simulink model "top_level_arch"  (R2025b)
settings: Solver=VariableStepAuto  StartTime=0.0  StopTime=10.0  RelTol=1e-3
undefined symbols (not defined in the file): D, L
(part 2 of 2)

== system top_level_arch/Manufacturing /Available Components/Propulsion ==
  Technology : Inport
  Supply Chain : Inport  Port=2
  Liquid Rocket : Subsystem  VariantControl=Ramjet1
      settings: PortSchema="{\"entries\":[{\"content\":{\"headerSize\":26,\"margin\":15,\"minimumSpacing\":25,\"sides\":[{\"content\":{},\"type\":\"ConnectorPlacement.EquallySpacedRectSide\",\"uuid\":\"e5d1d625-0a19-4884-bba9-d999bfe05807\"},{\"content\":{\"side\":\"RIGHT\"},\"type\":\"ConnectorPlacement.EquallySpacedRectSide\",\"uuid\":\"e3bc6884-47ae-4782-b1b3-7f6467d3ceaa\"},{\"content\":{\"side\":\"TOP\"},\"type\":\"ConnectorPlacement.EquallySpacedRectSide\",\"uuid\":\"e69a1f27-d2d1-47d9-a5bf-aefa7bba6fe5\"}]},\"type\":\"ConnectorPlacement.EquallySpacedConnector\",\"uuid\":\"2d31618d-9212-4cde-94a4-f40aa24b68df\"}],\"packageUris\":[\"http://schema.mathworks.com/mf0/Connector/R2020b\"],\"version\":\"1.0\"}"
  RDRE : Subsystem  VariantControl=true
      settings: PortSchema="{\"entries\":[{\"content\":{\"headerSize\":26,\"margin\":15,\"minimumSpacing\":25,\"sides\":[{\"content\":{},\"type\":\"ConnectorPlacement.EquallySpacedRectSide\",\"uuid\":\"e5d1d625-0a19-4884-bba9-d999bfe05807\"},{\"content\":{\"side\":\"RIGHT\"},\"type\":\"ConnectorPlacement.EquallySpacedRectSide\",\"uuid\":\"e3bc6884-47ae-4782-b1b3-7f6467d3ceaa\"},{\"content\":{\"side\":\"TOP\"},\"type\":\"ConnectorPlacement.EquallySpacedRectSide\",\"uuid\":\"e69a1f27-d2d1-47d9-a5bf-aefa7bba6fe5\"}]},\"type\":\"ConnectorPlacement.EquallySpacedConnector\",\"uuid\":\"2d31618d-9212-4cde-94a4-f40aa24b68df\"}],\"packageUris\":[\"http://schema.mathworks.com/mf0/Connector/R2020b\"],\"version\":\"1.0\"}"
  Ramjet : Subsystem  VariantControl=Turbojet1
      settings: PortSchema="{\"entries\":[{\"content\":{\"headerSize\":26,\"margin\":15,\"minimumSpacing\":25,\"sides\":[{\"content\":{},\"type\":\"ConnectorPlacement.EquallySpacedRectSide\",\"uuid\":\"e5d1d625-0a19-4884-bba9-d999bfe05807\"},{\"content\":{\"side\":\"RIGHT\"},\"type\":\"ConnectorPlacement.EquallySpacedRectSide\",\"uuid\":\"e3bc6884-47ae-4782-b1b3-7f6467d3ceaa\"},{\"content\":{\"side\":\"TOP\"},\"type\":\"ConnectorPlacement.EquallySpacedRectSide\",\"uuid\":\"e69a1f27-d2d1-47d9-a5bf-aefa7bba6fe5\"}]},\"type\":\"ConnectorPlacement.EquallySpacedConnector\",\"uuid\":\"2d31618d-9212-4cde-94a4-f40aa24b68df\"}],\"packageUris\":[\"http://schema.mathworks.com/mf0/Connector/R2020b\"],\"version\":\"1.0\"}"
  Solid Rocket : Subsystem  VariantControl=Liquid Rocket1
      settings: PortSchema="{\"entries\":[{\"content\":{\"headerSize\":26,\"margin\":15,\"minimumSpacing\":25,\"sides\":[{\"content\":{},\"type\":\"ConnectorPlacement.EquallySpacedRectSide\",\"uuid\":\"e5d1d625-0a19-4884-bba9-d999bfe05807\"},{\"content\":{\"side\":\"RIGHT\"},\"type\":\"ConnectorPlacement.EquallySpacedRectSide\",\"uuid\":\"e3bc6884-47ae-4782-b1b3-7f6467d3ceaa\"},{\"content\":{\"side\":\"TOP\"},\"type\":\"ConnectorPlacement.EquallySpacedRectSide\",\"uuid\":\"e69a1f27-d2d1-47d9-a5bf-aefa7bba6fe5\"}]},\"type\":\"ConnectorPlacement.EquallySpacedConnector\",\"uuid\":\"2d31618d-9212-4cde-94a4-f40aa24b68df\"}],\"packageUris\":[\"http://schema.mathworks.com/mf0/Connector/R2020b\"],\"version\":\"1.0\"}"
  Turbojet : Subsystem  VariantControl=false
      settings: PortSchema="{\"entries\":[{\"content\":{\"headerSize\":26,\"margin\":15,\"minimumSpacing\":25,\"sides\":[{\"content\":{},\"type\":\"ConnectorPlacement.EquallySpacedRectSide\",\"uuid\":\"e5d1d625-0a19-4884-bba9-d999bfe05807\"},{\"content\":{\"side\":\"RIGHT\"},\"type\":\"ConnectorPlacement.EquallySpacedRectSide\",\"uuid\":\"e3bc6884-47ae-4782-b1b3-7f6467d3ceaa\"},{\"content\":{\"side\":\"TOP\"},\"type\":\"ConnectorPlacement.EquallySpacedRectSide\",\"uuid\":\"e69a1f27-d2d1-47d9-a5bf-aefa7bba6fe5\"}]},\"type\":\"ConnectorPlacement.EquallySpacedConnector\",\"uuid\":\"2d31618d-9212-4cde-94a4-f40aa24b68df\"}],\"packageUris\":[\"http://schema.mathworks.com/mf0/Connector/R2020b\"],\"version\":\"1.0\"}"
  Propulsion Selection : Outport

== system top_level_arch/Manufacturing /Available Components/Software ==
  Bus Element In1 : Inport  PortName=Technology
  Bus Element In2 : Inport  Port=2  PortName=Supply Chain
  Bus Element Out1 : Outport  PortName=Software Vendor

== system top_level_arch/Scorpius Missile/Aerodynamics/Cylindrical ==

== system top_level_arch/Scorpius Missile/Aerodynamics/Delta Wing ==

== system top_level_arch/Scorpius Missile/Aerodynamics/Lifting Body ==

== system top_level_arch/Scorpius Missile/Configuration/External Hull ==
  Bus Element In1 : Inport  PortName=Assembly
  Bus Element Out1 : Outport  PortName=External Volume

== system top_level_arch/Scorpius Missile/Configuration/Folding Surfaces ==
  Assembly : Inport
  Folding Wings + Fins : Subsystem  VariantControl=false
      settings: PortSchema="{\"entries\":[{\"content\":{\"headerSize\":26,\"margin\":15,\"minimumSpacing\":25,\"sides\":[{\"content\":{},\"type\":\"ConnectorPlacement.EquallySpacedRectSide\",\"uuid\":\"ac629711-1768-428b-8fd7-79e4fe2b35a1\"},{\"content\":{\"side\":\"RIGHT\"},\"type\":\"ConnectorPlacement.EquallySpacedRectSide\",\"uuid\":\"b9c43ceb-249f-4c48-950c-a08a709e2313\"},{\"content\":{\"side\":\"TOP\"},\"type\":\"ConnectorPlacement.EquallySpacedRectSide\",\"uuid\":\"78a92a70-2dde-432d-9083-f129ee7bb076\"}]},\"type\":\"ConnectorPlacement.EquallySpacedConnector\",\"uuid\":\"b2b722ac-28c2-40e7-82d5-b0c5abc634fd\"}],\"packageUris\":[\"http://schema.mathworks.com/mf0/Connector/R2020b\"],\"version\":\"1.0\"}"
  Folding X-Fin : Subsystem  VariantControl=true
      settings: PortSchema="{\"entries\":[{\"content\":{\"headerSize\":26,\"margin\":15,\"minimumSpacing\":25,\"sides\":[{\"content\":{},\"type\":\"ConnectorPlacement.EquallySpacedRectSide\",\"uuid\":\"ac629711-1768-428b-8fd7-79e4fe2b35a1\"},{\"content\":{\"side\":\"RIGHT\"},\"type\":\"ConnectorPlacement.EquallySpacedRectSide\",\"uuid\":\"b9c43ceb-249f-4c48-950c-a08a709e2313\"},{\"content\":{\"side\":\"TOP\"},\"type\":\"ConnectorPlacement.EquallySpacedRectSide\",\"uuid\":\"78a92a70-2dde-432d-9083-f129ee7bb076\"}]},\"type\":\"ConnectorPlacement.EquallySpacedConnector\",\"uuid\":\"b2b722ac-28c2-40e7-82d5-b0c5abc634fd\"}],\"packageUris\":[\"http://schema.mathworks.com/mf0/Connector/R2020b\"],\"version\":\"1.0\"}"
  Launch Volume : Outport

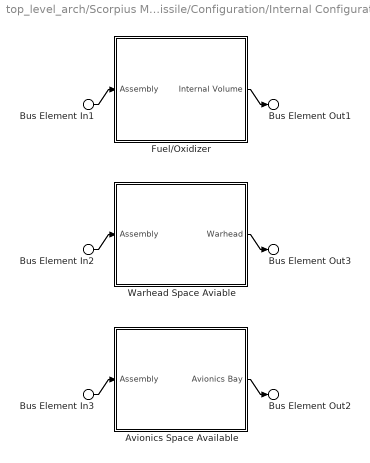
== system top_level_arch/Scorpius Missile/Configuration/Internal Configuration ==
  Bus Element In1 : Inport  PortName=Assembly
  Bus Element In2 : Inport  PortName=Assembly
  Bus Element In3 : Inport  PortName=Assembly
  Avionics Space Available : Subsystem
      settings: PortSchema="{\"entries\":[{\"content\":{\"headerSize\":26,\"margin\":15,\"minimumSpacing\":25,\"sides\":[{\"content\":{\"connectorIds\":[\"In1\"]},\"type\":\"ConnectorPlacement.EquallySpacedRectSide\",\"uuid\":\"dbfe6f62-bd81-4f2f-bf4a-ff0fc2c1733e\"},{\"content\":{\"connectorIds\":[\"Out1\"],\"side\":\"RIGHT\"},\"type\":\"ConnectorPlacement.EquallySpacedRectSide\",\"uuid\":\"15bb1ddd-14b3-4afc-89a1-8972fd4dab01\"},{\"content\":{\"side\":\"TOP\"},\"type\":\"ConnectorPlacement.EquallySpacedRectSide\",\"uuid\":\"d6068651-eb1a-4d26-9e8b-0135dded722b\"}]},\"type\":\"ConnectorPlacement.EquallySpacedConnector\",\"uuid\":\"074be2fd-c315-4aa4-8fc0-0402952ab401\"}],\"packageUris\":[\"http://schema.mathworks.com/mf0/Connector/R2020b\"],\"version\":\"1.0\"}"
  Fuel/Oxidizer : Subsystem
      settings: PortSchema="{\"entries\":[{\"content\":{\"headerSize\":26,\"margin\":15,\"minimumSpacing\":25,\"sides\":[{\"content\":{\"connectorIds\":[\"In1\"]},\"type\":\"ConnectorPlacement.EquallySpacedRectSide\",\"uuid\":\"dbfe6f62-bd81-4f2f-bf4a-ff0fc2c1733e\"},{\"content\":{\"connectorIds\":[\"Out1\"],\"side\":\"RIGHT\"},\"type\":\"ConnectorPlacement.EquallySpacedRectSide\",\"uuid\":\"15bb1ddd-14b3-4afc-89a1-8972fd4dab01\"},{\"content\":{\"side\":\"TOP\"},\"type\":\"ConnectorPlacement.EquallySpacedRectSide\",\"uuid\":\"d6068651-eb1a-4d26-9e8b-0135dded722b\"}]},\"type\":\"ConnectorPlacement.EquallySpacedConnector\",\"uuid\":\"074be2fd-c315-4aa4-8fc0-0402952ab401\"}],\"packageUris\":[\"http://schema.mathworks.com/mf0/Connector/R2020b\"],\"version\":\"1.0\"}"
  Warhead Space Aviable : Subsystem
      settings: PortSchema="{\"entries\":[{\"content\":{\"headerSize\":26,\"margin\":15,\"minimumSpacing\":25,\"sides\":[{\"content\":{\"connectorIds\":[\"In1\"]},\"type\":\"ConnectorPlacement.EquallySpacedRectSide\",\"uuid\":\"dbfe6f62-bd81-4f2f-bf4a-ff0fc2c1733e\"},{\"content\":{\"connectorIds\":[\"Out1\"],\"side\":\"RIGHT\"},\"type\":\"ConnectorPlacement.EquallySpacedRectSide\",\"uuid\":\"15bb1ddd-14b3-4afc-89a1-8972fd4dab01\"},{\"content\":{\"side\":\"TOP\"},\"type\":\"ConnectorPlacement.EquallySpacedRectSide\",\"uuid\":\"d6068651-eb1a-4d26-9e8b-0135dded722b\"}]},\"type\":\"ConnectorPlacement.EquallySpacedConnector\",\"uuid\":\"074be2fd-c315-4aa4-8fc0-0402952ab401\"}],\"packageUris\":[\"http://schema.mathworks.com/mf0/Connector/R2020b\"],\"version\":\"1.0\"}"
  Bus Element Out1 : Outport  PortName=Internal Volume
  Bus Element Out3 : Outport  Port=2  PortName=Warhead
  Bus Element Out2 : Outport  Port=3  PortName=Avionics Bay
  wires:
  Bus Element In1/1 -> Fuel/Oxidizer/1(Assembly)
  Bus Element In2/1 -> Warhead Space Aviable/1(Assembly)
  Bus Element In3/1 -> Avionics Space Available/1(Assembly)
  Fuel/Oxidizer/1(Internal Volume) -> Bus Element Out1/1
  Warhead Space Aviable/1(Warhead) -> Bus Element Out3/1
  Avionics Space Available/1(Avionics Bay) -> Bus Element Out2/1

== system top_level_arch/Scorpius Missile/Propulsion/Fuel//Oxidizer Tank ==
  Bus Element In1 : Inport  PortName=Internal Volume
  Bus Element Out1 : Outport  PortName=Fuel Capacity

== system top_level_arch/Scorpius Missile/Propulsion/RDRE ==
  Bus Element In1 : Inport  PortName=Fuel Capacity
  Bus Element Out2 : Outport  PortName=Supersonic Cruise
  Bus Element Out1 : Outport  Port=2  PortName=Fuel Consumption
  Bus Element Out3 : Outport  Port=3  PortName=Thrust

== system top_level_arch/Scorpius Missile/Trajectory/Approach ==
  Avionics Bay : Inport
  L/D : Inport  Port=2
  Range : Inport  Port=3
  Direct Dive : Subsystem  VariantControl=true  mask{DiveRange=[]}
      settings: PortSchema="{\"entries\":[{\"content\":{\"headerSize\":26,\"margin\":15,\"minimumSpacing\":25,\"sides\":[{\"content\":{},\"type\":\"ConnectorPlacement.EquallySpacedRectSide\",\"uuid\":\"ac629711-1768-428b-8fd7-79e4fe2b35a1\"},{\"content\":{\"side\":\"RIGHT\"},\"type\":\"ConnectorPlacement.EquallySpacedRectSide\",\"uuid\":\"b9c43ceb-249f-4c48-950c-a08a709e2313\"},{\"content\":{\"side\":\"TOP\"},\"type\":\"ConnectorPlacement.EquallySpacedRectSide\",\"uuid\":\"78a92a70-2dde-432d-9083-f129ee7bb076\"}]},\"type\":\"ConnectorPlacement.EquallySpacedConnector\",\"uuid\":\"b2b722ac-28c2-40e7-82d5-b0c5abc634fd\"}],\"packageUris\":[\"http://schema.mathworks.com/mf0/Connector/R2020b\"],\"version\":\"1.0\"}"
  Low Level Ingress : Subsystem  VariantControl=false  mask{LLIRange=[]}
      settings: PortSchema="{\"entries\":[{\"content\":{\"headerSize\":26,\"margin\":15,\"minimumSpacing\":25,\"sides\":[{\"content\":{},\"type\":\"ConnectorPlacement.EquallySpacedRectSide\",\"uuid\":\"ac629711-1768-428b-8fd7-79e4fe2b35a1\"},{\"content\":{\"side\":\"RIGHT\"},\"type\":\"ConnectorPlacement.EquallySpacedRectSide\",\"uuid\":\"b9c43ceb-249f-4c48-950c-a08a709e2313\"},{\"content\":{\"side\":\"TOP\"},\"type\":\"ConnectorPlacement.EquallySpacedRectSide\",\"uuid\":\"78a92a70-2dde-432d-9083-f129ee7bb076\"}]},\"type\":\"ConnectorPlacement.EquallySpacedConnector\",\"uuid\":\"b2b722ac-28c2-40e7-82d5-b0c5abc634fd\"}],\"packageUris\":[\"http://schema.mathworks.com/mf0/Connector/R2020b\"],\"version\":\"1.0\"}"
  Approach Phase : Outport
  Target Approach : Outport  Port=2

== system top_level_arch/Scorpius Missile/Trajectory/Climb ==
  Bus Element In1 : Inport  PortName=L/D
  Bus Element In2 : Inport  Port=2  PortName=Range
  Bus Element In3 : Inport  Port=3  PortName=Thrust
  Bus Element Out1 : Outport  PortName=Climb Phase

== system top_level_arch/Scorpius Missile/Trajectory/Cruise ==
  Bus Element In1 : Inport  PortName=L/D
  Bus Element In2 : Inport  Port=2  PortName=Range
  Bus Element In3 : Inport  Port=3  PortName=Thrust
  Bus Element Out1 : Outport  PortName=Cruise Phase

== system top_level_arch/Scorpius Missile/Trajectory/Glide ==
  Bus Element In1 : Inport  PortName=L/D
  Bus Element Out1 : Outport  PortName=Glide Phase

== system top_level_arch/Manufacturing /Available Components/Avionics Package/Air Data System ==
  Technology : Inport
  Supply Chain : Inport  Port=2
  Flush Air Data System : Subsystem  VariantControl=false
      settings: PortSchema="{\"entries\":[{\"content\":{\"headerSize\":26,\"margin\":15,\"minimumSpacing\":25,\"sides\":[{\"content\":{},\"type\":\"ConnectorPlacement.EquallySpacedRectSide\",\"uuid\":\"ac629711-1768-428b-8fd7-79e4fe2b35a1\"},{\"content\":{\"side\":\"RIGHT\"},\"type\":\"ConnectorPlacement.EquallySpacedRectSide\",\"uuid\":\"b9c43ceb-249f-4c48-950c-a08a709e2313\"},{\"content\":{\"side\":\"TOP\"},\"type\":\"ConnectorPlacement.EquallySpacedRectSide\",\"uuid\":\"78a92a70-2dde-432d-9083-f129ee7bb076\"}]},\"type\":\"ConnectorPlacement.EquallySpacedConnector\",\"uuid\":\"b2b722ac-28c2-40e7-82d5-b0c5abc634fd\"}],\"packageUris\":[\"http://schema.mathworks.com/mf0/Connector/R2020b\"],\"version\":\"1.0\"}"
  Pitot Tube : Subsystem  VariantControl=true
      settings: PortSchema="{\"entries\":[{\"content\":{\"headerSize\":26,\"margin\":15,\"minimumSpacing\":25,\"sides\":[{\"content\":{},\"type\":\"ConnectorPlacement.EquallySpacedRectSide\",\"uuid\":\"ac629711-1768-428b-8fd7-79e4fe2b35a1\"},{\"content\":{\"side\":\"RIGHT\"},\"type\":\"ConnectorPlacement.EquallySpacedRectSide\",\"uuid\":\"b9c43ceb-249f-4c48-950c-a08a709e2313\"},{\"content\":{\"side\":\"TOP\"},\"type\":\"ConnectorPlacement.EquallySpacedRectSide\",\"uuid\":\"78a92a70-2dde-432d-9083-f129ee7bb076\"}]},\"type\":\"ConnectorPlacement.EquallySpacedConnector\",\"uuid\":\"b2b722ac-28c2-40e7-82d5-b0c5abc634fd\"}],\"packageUris\":[\"http://schema.mathworks.com/mf0/Connector/R2020b\"],\"version\":\"1.0\"}"
  Air Data Selection : Outport

== system top_level_arch/Manufacturing /Available Components/Avionics Package/Battery ==
  Technology : Inport
  Supply Chain : Inport  Port=2
  Battery 1 : Subsystem  VariantControl=true
      settings: PortSchema="{\"entries\":[{\"content\":{\"headerSize\":26,\"margin\":15,\"minimumSpacing\":25,\"sides\":[{\"content\":{},\"type\":\"ConnectorPlacement.EquallySpacedRectSide\",\"uuid\":\"ac629711-1768-428b-8fd7-79e4fe2b35a1\"},{\"content\":{\"side\":\"RIGHT\"},\"type\":\"ConnectorPlacement.EquallySpacedRectSide\",\"uuid\":\"b9c43ceb-249f-4c48-950c-a08a709e2313\"},{\"content\":{\"side\":\"TOP\"},\"type\":\"ConnectorPlacement.EquallySpacedRectSide\",\"uuid\":\"78a92a70-2dde-432d-9083-f129ee7bb076\"}]},\"type\":\"ConnectorPlacement.EquallySpacedConnector\",\"uuid\":\"b2b722ac-28c2-40e7-82d5-b0c5abc634fd\"}],\"packageUris\":[\"http://schema.mathworks.com/mf0/Connector/R2020b\"],\"version\":\"1.0\"}"
  Battery 2 : Subsystem  VariantControl=false
      settings: PortSchema="{\"entries\":[{\"content\":{\"headerSize\":26,\"margin\":15,\"minimumSpacing\":25,\"sides\":[{\"content\":{},\"type\":\"ConnectorPlacement.EquallySpacedRectSide\",\"uuid\":\"ac629711-1768-428b-8fd7-79e4fe2b35a1\"},{\"content\":{\"side\":\"RIGHT\"},\"type\":\"ConnectorPlacement.EquallySpacedRectSide\",\"uuid\":\"b9c43ceb-249f-4c48-950c-a08a709e2313\"},{\"content\":{\"side\":\"TOP\"},\"type\":\"ConnectorPlacement.EquallySpacedRectSide\",\"uuid\":\"78a92a70-2dde-432d-9083-f129ee7bb076\"}]},\"type\":\"ConnectorPlacement.EquallySpacedConnector\",\"uuid\":\"b2b722ac-28c2-40e7-82d5-b0c5abc634fd\"}],\"packageUris\":[\"http://schema.mathworks.com/mf0/Connector/R2020b\"],\"version\":\"1.0\"}"
  Battery Selection : Outport

== system top_level_arch/Manufacturing /Available Components/Avionics Package/Guidance Package ==
  Target Approach : Inport
  Technology : Inport  Port=2
  Supply Chain : Inport  Port=3
  Dive Package : Subsystem  VariantControl=true
      settings: PortSchema="{\"entries\":[{\"content\":{\"headerSize\":26,\"margin\":15,\"minimumSpacing\":25,\"sides\":[{\"content\":{},\"type\":\"ConnectorPlacement.EquallySpacedRectSide\",\"uuid\":\"ac629711-1768-428b-8fd7-79e4fe2b35a1\"},{\"content\":{\"side\":\"RIGHT\"},\"type\":\"ConnectorPlacement.EquallySpacedRectSide\",\"uuid\":\"b9c43ceb-249f-4c48-950c-a08a709e2313\"},{\"content\":{\"side\":\"TOP\"},\"type\":\"ConnectorPlacement.EquallySpacedRectSide\",\"uuid\":\"78a92a70-2dde-432d-9083-f129ee7bb076\"}]},\"type\":\"ConnectorPlacement.EquallySpacedConnector\",\"uuid\":\"b2b722ac-28c2-40e7-82d5-b0c5abc634fd\"}],\"packageUris\":[\"http://schema.mathworks.com/mf0/Connector/R2020b\"],\"version\":\"1.0\"}"
  LLI Package : Subsystem  VariantControl=false
      settings: PortSchema="{\"entries\":[{\"content\":{\"headerSize\":26,\"margin\":15,\"minimumSpacing\":25,\"sides\":[{\"content\":{},\"type\":\"ConnectorPlacement.EquallySpacedRectSide\",\"uuid\":\"ac629711-1768-428b-8fd7-79e4fe2b35a1\"},{\"content\":{\"side\":\"RIGHT\"},\"type\":\"ConnectorPlacement.EquallySpacedRectSide\",\"uuid\":\"b9c43ceb-249f-4c48-950c-a08a709e2313\"},{\"content\":{\"side\":\"TOP\"},\"type\":\"ConnectorPlacement.EquallySpacedRectSide\",\"uuid\":\"78a92a70-2dde-432d-9083-f129ee7bb076\"}]},\"type\":\"ConnectorPlacement.EquallySpacedConnector\",\"uuid\":\"b2b722ac-28c2-40e7-82d5-b0c5abc634fd\"}],\"packageUris\":[\"http://schema.mathworks.com/mf0/Connector/R2020b\"],\"version\":\"1.0\"}"
  Guidance Selection : Outport

== system top_level_arch/Manufacturing /Available Components/Avionics Package/Target Identification//Tracking ==
  Bus Element In1 : Inport  PortName=Technology
  Bus Element In2 : Inport  Port=2  PortName=Supply Chain
  IR Camera : Subsystem
      settings: PortSchema="{\"entries\":[{\"content\":{\"headerSize\":26,\"margin\":15,\"minimumSpacing\":25,\"sides\":[{\"content\":{},\"type\":\"ConnectorPlacement.EquallySpacedRectSide\",\"uuid\":\"acffec25-5f7e-46a6-bfc3-7ef631e1638e\"},{\"content\":{\"side\":\"RIGHT\"},\"type\":\"ConnectorPlacement.EquallySpacedRectSide\",\"uuid\":\"2e9e2c31-11a0-4694-98ae-75af4a65f270\"},{\"content\":{\"side\":\"TOP\"},\"type\":\"ConnectorPlacement.EquallySpacedRectSide\",\"uuid\":\"496cd80b-0660-4c9b-9e86-ee3459eee66e\"}]},\"type\":\"ConnectorPlacement.EquallySpacedConnector\",\"uuid\":\"b09bcaf7-bc67-4c5f-bdb5-a74881794e47\"}],\"packageUris\":[\"http://schema.mathworks.com/mf0/Connector/R2020b\"],\"version\":\"1.0\"}"
  Radar Seeker : Subsystem
      settings: PortSchema="{\"entries\":[{\"content\":{\"headerSize\":26,\"margin\":15,\"minimumSpacing\":25,\"sides\":[{\"content\":{},\"type\":\"ConnectorPlacement.EquallySpacedRectSide\",\"uuid\":\"acffec25-5f7e-46a6-bfc3-7ef631e1638e\"},{\"content\":{\"side\":\"RIGHT\"},\"type\":\"ConnectorPlacement.EquallySpacedRectSide\",\"uuid\":\"2e9e2c31-11a0-4694-98ae-75af4a65f270\"},{\"content\":{\"side\":\"TOP\"},\"type\":\"ConnectorPlacement.EquallySpacedRectSide\",\"uuid\":\"496cd80b-0660-4c9b-9e86-ee3459eee66e\"}]},\"type\":\"ConnectorPlacement.EquallySpacedConnector\",\"uuid\":\"b09bcaf7-bc67-4c5f-bdb5-a74881794e47\"}],\"packageUris\":[\"http://schema.mathworks.com/mf0/Connector/R2020b\"],\"version\":\"1.0\"}"
  Bus Element Out1 : Outport  PortName=Tracking Selection

== system top_level_arch/Manufacturing /Available Components/Avionics Package/Viewport ==
  Technology : Inport
  Supply Chain : Inport  Port=2
  ALON : Subsystem  VariantControl=false
      settings: PortSchema="{\"entries\":[{\"content\":{\"headerSize\":26,\"margin\":15,\"minimumSpacing\":25,\"sides\":[{\"content\":{},\"type\":\"ConnectorPlacement.EquallySpacedRectSide\",\"uuid\":\"14d9ea52-85a6-4fb4-904c-7b9934a78a94\"},{\"content\":{\"side\":\"RIGHT\"},\"type\":\"ConnectorPlacement.EquallySpacedRectSide\",\"uuid\":\"864c2340-4ef1-4369-9a4a-c7cd50a8f0c1\"},{\"content\":{\"side\":\"TOP\"},\"type\":\"ConnectorPlacement.EquallySpacedRectSide\",\"uuid\":\"28f02aed-ac94-4b4c-b7bc-b8c70f1f15b4\"}]},\"type\":\"ConnectorPlacement.EquallySpacedConnector\",\"uuid\":\"ad27087a-bf5d-4673-98c0-ee0a7adf1b04\"}],\"packageUris\":[\"http://schema.mathworks.com/mf0/Connector/R2020b\"],\"version\":\"1.0\"}"
  Sapphire : Subsystem  VariantControl=true
      settings: PortSchema="{\"entries\":[{\"content\":{\"headerSize\":26,\"margin\":15,\"minimumSpacing\":25,\"sides\":[{\"content\":{},\"type\":\"ConnectorPlacement.EquallySpacedRectSide\",\"uuid\":\"14d9ea52-85a6-4fb4-904c-7b9934a78a94\"},{\"content\":{\"side\":\"RIGHT\"},\"type\":\"ConnectorPlacement.EquallySpacedRectSide\",\"uuid\":\"864c2340-4ef1-4369-9a4a-c7cd50a8f0c1\"},{\"content\":{\"side\":\"TOP\"},\"type\":\"ConnectorPlacement.EquallySpacedRectSide\",\"uuid\":\"28f02aed-ac94-4b4c-b7bc-b8c70f1f15b4\"}]},\"type\":\"ConnectorPlacement.EquallySpacedConnector\",\"uuid\":\"ad27087a-bf5d-4673-98c0-ee0a7adf1b04\"}],\"packageUris\":[\"http://schema.mathworks.com/mf0/Connector/R2020b\"],\"version\":\"1.0\"}"
  Viewport Selection : Outport

== system top_level_arch/Manufacturing /Available Components/Materials/Structural Material ==
  Heating : Inport
  Supply Chain : Inport  Port=2
  ALON : Subsystem  VariantControl=Titantium1
      settings: PortSchema="{\"entries\":[{\"content\":{\"headerSize\":26,\"margin\":15,\"minimumSpacing\":25,\"sides\":[{\"content\":{},\"type\":\"ConnectorPlacement.EquallySpacedRectSide\",\"uuid\":\"e5d1d625-0a19-4884-bba9-d999bfe05807\"},{\"content\":{\"side\":\"RIGHT\"},\"type\":\"ConnectorPlacement.EquallySpacedRectSide\",\"uuid\":\"e3bc6884-47ae-4782-b1b3-7f6467d3ceaa\"},{\"content\":{\"side\":\"TOP\"},\"type\":\"ConnectorPlacement.EquallySpacedRectSide\",\"uuid\":\"e69a1f27-d2d1-47d9-a5bf-aefa7bba6fe5\"}]},\"type\":\"ConnectorPlacement.EquallySpacedConnector\",\"uuid\":\"2d31618d-9212-4cde-94a4-f40aa24b68df\"}],\"packageUris\":[\"http://schema.mathworks.com/mf0/Connector/R2020b\"],\"version\":\"1.0\"}"
  Inconel : Subsystem  VariantControl=false
      settings: PortSchema="{\"entries\":[{\"content\":{\"headerSize\":26,\"margin\":15,\"minimumSpacing\":25,\"sides\":[{\"content\":{},\"type\":\"ConnectorPlacement.EquallySpacedRectSide\",\"uuid\":\"e5d1d625-0a19-4884-bba9-d999bfe05807\"},{\"content\":{\"side\":\"RIGHT\"},\"type\":\"ConnectorPlacement.EquallySpacedRectSide\",\"uuid\":\"e3bc6884-47ae-4782-b1b3-7f6467d3ceaa\"},{\"content\":{\"side\":\"TOP\"},\"type\":\"ConnectorPlacement.EquallySpacedRectSide\",\"uuid\":\"e69a1f27-d2d1-47d9-a5bf-aefa7bba6fe5\"}]},\"type\":\"ConnectorPlacement.EquallySpacedConnector\",\"uuid\":\"2d31618d-9212-4cde-94a4-f40aa24b68df\"}],\"packageUris\":[\"http://schema.mathworks.com/mf0/Connector/R2020b\"],\"version\":\"1.0\"}"
  Stainless Steel : Subsystem  VariantControl=true
      settings: PortSchema="{\"entries\":[{\"content\":{\"headerSize\":26,\"margin\":15,\"minimumSpacing\":25,\"sides\":[{\"content\":{},\"type\":\"ConnectorPlacement.EquallySpacedRectSide\",\"uuid\":\"e5d1d625-0a19-4884-bba9-d999bfe05807\"},{\"content\":{\"side\":\"RIGHT\"},\"type\":\"ConnectorPlacement.EquallySpacedRectSide\",\"uuid\":\"e3bc6884-47ae-4782-b1b3-7f6467d3ceaa\"},{\"content\":{\"side\":\"TOP\"},\"type\":\"ConnectorPlacement.EquallySpacedRectSide\",\"uuid\":\"e69a1f27-d2d1-47d9-a5bf-aefa7bba6fe5\"}]},\"type\":\"ConnectorPlacement.EquallySpacedConnector\",\"uuid\":\"2d31618d-9212-4cde-94a4-f40aa24b68df\"}],\"packageUris\":[\"http://schema.mathworks.com/mf0/Connector/R2020b\"],\"version\":\"1.0\"}"
  Titantium : Subsystem  VariantControl=Inconel1
      settings: PortSchema="{\"entries\":[{\"content\":{\"headerSize\":26,\"margin\":15,\"minimumSpacing\":25,\"sides\":[{\"content\":{},\"type\":\"ConnectorPlacement.EquallySpacedRectSide\",\"uuid\":\"e5d1d625-0a19-4884-bba9-d999bfe05807\"},{\"content\":{\"side\":\"RIGHT\"},\"type\":\"ConnectorPlacement.EquallySpacedRectSide\",\"uuid\":\"e3bc6884-47ae-4782-b1b3-7f6467d3ceaa\"},{\"content\":{\"side\":\"TOP\"},\"type\":\"ConnectorPlacement.EquallySpacedRectSide\",\"uuid\":\"e69a1f27-d2d1-47d9-a5bf-aefa7bba6fe5\"}]},\"type\":\"ConnectorPlacement.EquallySpacedConnector\",\"uuid\":\"2d31618d-9212-4cde-94a4-f40aa24b68df\"}],\"packageUris\":[\"http://schema.mathworks.com/mf0/Connector/R2020b\"],\"version\":\"1.0\"}"
  Structural Materials Selection : Outport

== system top_level_arch/Manufacturing /Available Components/Materials/Thermal Material ==
  Bus Element In2 : Inport  PortName=Heating
  Bus Element In1 : Inport  Port=2  PortName=Supply Chain
  AeroTape : Subsystem
      settings: PortSchema="{\"entries\":[{\"content\":{\"headerSize\":26,\"margin\":15,\"minimumSpacing\":25,\"sides\":[{\"content\":{},\"type\":\"ConnectorPlacement.EquallySpacedRectSide\",\"uuid\":\"32e1f4e9-0392-4c12-9305-55f9b62cf007\"},{\"content\":{\"side\":\"RIGHT\"},\"type\":\"ConnectorPlacement.EquallySpacedRectSide\",\"uuid\":\"8bf8c952-69c8-496e-947f-24d197d632d3\"},{\"content\":{\"side\":\"TOP\"},\"type\":\"ConnectorPlacement.EquallySpacedRectSide\",\"uuid\":\"adf3e777-baf5-48a6-a5b4-f0ede588bd33\"}]},\"type\":\"ConnectorPlacement.EquallySpacedConnector\",\"uuid\":\"9ec8f034-0877-461e-a570-0bf1a23861f1\"}],\"packageUris\":[\"http://schema.mathworks.com/mf0/Connector/R2020b\"],\"version\":\"1.0\"}"
  Carbon Ablators : Subsystem
      settings: PortSchema="{\"entries\":[{\"content\":{\"headerSize\":26,\"margin\":15,\"minimumSpacing\":25,\"sides\":[{\"content\":{},\"type\":\"ConnectorPlacement.EquallySpacedRectSide\",\"uuid\":\"32e1f4e9-0392-4c12-9305-55f9b62cf007\"},{\"content\":{\"side\":\"RIGHT\"},\"type\":\"ConnectorPlacement.EquallySpacedRectSide\",\"uuid\":\"8bf8c952-69c8-496e-947f-24d197d632d3\"},{\"content\":{\"side\":\"TOP\"},\"type\":\"ConnectorPlacement.EquallySpacedRectSide\",\"uuid\":\"adf3e777-baf5-48a6-a5b4-f0ede588bd33\"}]},\"type\":\"ConnectorPlacement.EquallySpacedConnector\",\"uuid\":\"9ec8f034-0877-461e-a570-0bf1a23861f1\"}],\"packageUris\":[\"http://schema.mathworks.com/mf0/Connector/R2020b\"],\"version\":\"1.0\"}"
  Bus Element Out1 : Outport  PortName=Thermal Materials Selection

== system top_level_arch/Manufacturing /Available Components/Propulsion/Liquid Rocket ==

== system top_level_arch/Manufacturing /Available Components/Propulsion/RDRE ==

== system top_level_arch/Manufacturing /Available Components/Propulsion/Ramjet ==

== system top_level_arch/Manufacturing /Available Components/Propulsion/Solid Rocket ==

== system top_level_arch/Manufacturing /Available Components/Propulsion/Turbojet ==

== system top_level_arch/Scorpius Missile/Configuration/Folding Surfaces/Folding Wings + Fins ==

== system top_level_arch/Scorpius Missile/Configuration/Folding Surfaces/Folding X-Fin ==

== system top_level_arch/Scorpius Missile/Configuration/Internal Configuration/Avionics Space Available ==
  Bus Element In1 : Inport  PortName=Assembly
  Bus Element Out1 : Outport  PortName=Avionics Bay

== system top_level_arch/Scorpius Missile/Configuration/Internal Configuration/Fuel//Oxidizer ==
  Bus Element In1 : Inport  PortName=Assembly
  Bus Element Out1 : Outport  PortName=Internal Volume

== system top_level_arch/Scorpius Missile/Configuration/Internal Configuration/Warhead Space Aviable ==
  Bus Element In1 : Inport  PortName=Assembly
  Bus Element Out1 : Outport  PortName=Warhead

== system top_level_arch/Scorpius Missile/Trajectory/Approach/Direct Dive ==

== system top_level_arch/Scorpius Missile/Trajectory/Approach/Low Level Ingress ==

== system top_level_arch/Manufacturing /Available Components/Avionics Package/Air Data System/Flush Air Data System ==

== system top_level_arch/Manufacturing /Available Components/Avionics Package/Air Data System/Pitot Tube ==

== system top_level_arch/Manufacturing /Available Components/Avionics Package/Battery/Battery 1 ==

== system top_level_arch/Manufacturing /Available Components/Avionics Package/Battery/Battery 2 ==

== system top_level_arch/Manufacturing /Available Components/Avionics Package/Guidance Package/Dive Package ==
  DISMAC : Subsystem
      settings: PortSchema="{\"entries\":[{\"content\":{\"headerSize\":26,\"margin\":15,\"minimumSpacing\":25,\"sides\":[{\"content\":{},\"type\":\"ConnectorPlacement.EquallySpacedRectSide\",\"uuid\":\"f725402c-10b5-4b82-85cc-51bef2710ba8\"},{\"content\":{\"side\":\"RIGHT\"},\"type\":\"ConnectorPlacement.EquallySpacedRectSide\",\"uuid\":\"62fc519a-e2d1-4367-b68f-022d97ba9f16\"},{\"content\":{\"side\":\"TOP\"},\"type\":\"ConnectorPlacement.EquallySpacedRectSide\",\"uuid\":\"613b120d-3cdc-496e-8a51-984c64e3d49e\"}]},\"type\":\"ConnectorPlacement.EquallySpacedConnector\",\"uuid\":\"aaea6f75-d808-4e3f-996d-2fe6c7697c49\"}],\"packageUris\":[\"http://schema.mathworks.com/mf0/Connector/R2020b\"],\"version\":\"1.0\"}"
  GPS : Subsystem
      settings: PortSchema="{\"entries\":[{\"content\":{\"headerSize\":26,\"margin\":15,\"minimumSpacing\":25,\"sides\":[{\"content\":{},\"type\":\"ConnectorPlacement.EquallySpacedRectSide\",\"uuid\":\"f725402c-10b5-4b82-85cc-51bef2710ba8\"},{\"content\":{\"side\":\"RIGHT\"},\"type\":\"ConnectorPlacement.EquallySpacedRectSide\",\"uuid\":\"62fc519a-e2d1-4367-b68f-022d97ba9f16\"},{\"content\":{\"side\":\"TOP\"},\"type\":\"ConnectorPlacement.EquallySpacedRectSide\",\"uuid\":\"613b120d-3cdc-496e-8a51-984c64e3d49e\"}]},\"type\":\"ConnectorPlacement.EquallySpacedConnector\",\"uuid\":\"aaea6f75-d808-4e3f-996d-2fe6c7697c49\"}],\"packageUris\":[\"http://schema.mathworks.com/mf0/Connector/R2020b\"],\"version\":\"1.0\"}"
  IMU : Subsystem
      settings: PortSchema="{\"entries\":[{\"content\":{\"headerSize\":26,\"margin\":15,\"minimumSpacing\":25,\"sides\":[{\"content\":{},\"type\":\"ConnectorPlacement.EquallySpacedRectSide\",\"uuid\":\"f725402c-10b5-4b82-85cc-51bef2710ba8\"},{\"content\":{\"side\":\"RIGHT\"},\"type\":\"ConnectorPlacement.EquallySpacedRectSide\",\"uuid\":\"62fc519a-e2d1-4367-b68f-022d97ba9f16\"},{\"content\":{\"side\":\"TOP\"},\"type\":\"ConnectorPlacement.EquallySpacedRectSide\",\"uuid\":\"613b120d-3cdc-496e-8a51-984c64e3d49e\"}]},\"type\":\"ConnectorPlacement.EquallySpacedConnector\",\"uuid\":\"aaea6f75-d808-4e3f-996d-2fe6c7697c49\"}],\"packageUris\":[\"http://schema.mathworks.com/mf0/Connector/R2020b\"],\"version\":\"1.0\"}"
  STAR Tracker : Subsystem
      settings: PortSchema="{\"entries\":[{\"content\":{\"headerSize\":26,\"margin\":15,\"minimumSpacing\":25,\"sides\":[{\"content\":{},\"type\":\"ConnectorPlacement.EquallySpacedRectSide\",\"uuid\":\"f725402c-10b5-4b82-85cc-51bef2710ba8\"},{\"content\":{\"side\":\"RIGHT\"},\"type\":\"ConnectorPlacement.EquallySpacedRectSide\",\"uuid\":\"62fc519a-e2d1-4367-b68f-022d97ba9f16\"},{\"content\":{\"side\":\"TOP\"},\"type\":\"ConnectorPlacement.EquallySpacedRectSide\",\"uuid\":\"613b120d-3cdc-496e-8a51-984c64e3d49e\"}]},\"type\":\"ConnectorPlacement.EquallySpacedConnector\",\"uuid\":\"aaea6f75-d808-4e3f-996d-2fe6c7697c49\"}],\"packageUris\":[\"http://schema.mathworks.com/mf0/Connector/R2020b\"],\"version\":\"1.0\"}"

== system top_level_arch/Manufacturing /Available Components/Avionics Package/Guidance Package/LLI Package ==
  DISMAC : Subsystem
      settings: PortSchema="{\"entries\":[{\"content\":{\"headerSize\":26,\"margin\":15,\"minimumSpacing\":25,\"sides\":[{\"content\":{},\"type\":\"ConnectorPlacement.EquallySpacedRectSide\",\"uuid\":\"f725402c-10b5-4b82-85cc-51bef2710ba8\"},{\"content\":{\"side\":\"RIGHT\"},\"type\":\"ConnectorPlacement.EquallySpacedRectSide\",\"uuid\":\"62fc519a-e2d1-4367-b68f-022d97ba9f16\"},{\"content\":{\"side\":\"TOP\"},\"type\":\"ConnectorPlacement.EquallySpacedRectSide\",\"uuid\":\"613b120d-3cdc-496e-8a51-984c64e3d49e\"}]},\"type\":\"ConnectorPlacement.EquallySpacedConnector\",\"uuid\":\"aaea6f75-d808-4e3f-996d-2fe6c7697c49\"}],\"packageUris\":[\"http://schema.mathworks.com/mf0/Connector/R2020b\"],\"version\":\"1.0\"}"
  GPS : Subsystem
      settings: PortSchema="{\"entries\":[{\"content\":{\"headerSize\":26,\"margin\":15,\"minimumSpacing\":25,\"sides\":[{\"content\":{},\"type\":\"ConnectorPlacement.EquallySpacedRectSide\",\"uuid\":\"f725402c-10b5-4b82-85cc-51bef2710ba8\"},{\"content\":{\"side\":\"RIGHT\"},\"type\":\"ConnectorPlacement.EquallySpacedRectSide\",\"uuid\":\"62fc519a-e2d1-4367-b68f-022d97ba9f16\"},{\"content\":{\"side\":\"TOP\"},\"type\":\"ConnectorPlacement.EquallySpacedRectSide\",\"uuid\":\"613b120d-3cdc-496e-8a51-984c64e3d49e\"}]},\"type\":\"ConnectorPlacement.EquallySpacedConnector\",\"uuid\":\"aaea6f75-d808-4e3f-996d-2fe6c7697c49\"}],\"packageUris\":[\"http://schema.mathworks.com/mf0/Connector/R2020b\"],\"version\":\"1.0\"}"
  IMU : Subsystem
      settings: PortSchema="{\"entries\":[{\"content\":{\"headerSize\":26,\"margin\":15,\"minimumSpacing\":25,\"sides\":[{\"content\":{},\"type\":\"ConnectorPlacement.EquallySpacedRectSide\",\"uuid\":\"f725402c-10b5-4b82-85cc-51bef2710ba8\"},{\"content\":{\"side\":\"RIGHT\"},\"type\":\"ConnectorPlacement.EquallySpacedRectSide\",\"uuid\":\"62fc519a-e2d1-4367-b68f-022d97ba9f16\"},{\"content\":{\"side\":\"TOP\"},\"type\":\"ConnectorPlacement.EquallySpacedRectSide\",\"uuid\":\"613b120d-3cdc-496e-8a51-984c64e3d49e\"}]},\"type\":\"ConnectorPlacement.EquallySpacedConnector\",\"uuid\":\"aaea6f75-d808-4e3f-996d-2fe6c7697c49\"}],\"packageUris\":[\"http://schema.mathworks.com/mf0/Connector/R2020b\"],\"version\":\"1.0\"}"
  STAR Tracker : Subsystem
      settings: PortSchema="{\"entries\":[{\"content\":{\"headerSize\":26,\"margin\":15,\"minimumSpacing\":25,\"sides\":[{\"content\":{},\"type\":\"ConnectorPlacement.EquallySpacedRectSide\",\"uuid\":\"f725402c-10b5-4b82-85cc-51bef2710ba8\"},{\"content\":{\"side\":\"RIGHT\"},\"type\":\"ConnectorPlacement.EquallySpacedRectSide\",\"uuid\":\"62fc519a-e2d1-4367-b68f-022d97ba9f16\"},{\"content\":{\"side\":\"TOP\"},\"type\":\"ConnectorPlacement.EquallySpacedRectSide\",\"uuid\":\"613b120d-3cdc-496e-8a51-984c64e3d49e\"}]},\"type\":\"ConnectorPlacement.EquallySpacedConnector\",\"uuid\":\"aaea6f75-d808-4e3f-996d-2fe6c7697c49\"}],\"packageUris\":[\"http://schema.mathworks.com/mf0/Connector/R2020b\"],\"version\":\"1.0\"}"
  TARCOM : Subsystem
      settings: PortSchema="{\"entries\":[{\"content\":{\"headerSize\":26,\"margin\":15,\"minimumSpacing\":25,\"sides\":[{\"content\":{},\"type\":\"ConnectorPlacement.EquallySpacedRectSide\",\"uuid\":\"f725402c-10b5-4b82-85cc-51bef2710ba8\"},{\"content\":{\"side\":\"RIGHT\"},\"type\":\"ConnectorPlacement.EquallySpacedRectSide\",\"uuid\":\"62fc519a-e2d1-4367-b68f-022d97ba9f16\"},{\"content\":{\"side\":\"TOP\"},\"type\":\"ConnectorPlacement.EquallySpacedRectSide\",\"uuid\":\"613b120d-3cdc-496e-8a51-984c64e3d49e\"}]},\"type\":\"ConnectorPlacement.EquallySpacedConnector\",\"uuid\":\"aaea6f75-d808-4e3f-996d-2fe6c7697c49\"}],\"packageUris\":[\"http://schema.mathworks.com/mf0/Connector/R2020b\"],\"version\":\"1.0\"}"

== system top_level_arch/Manufacturing /Available Components/Avionics Package/Target Identification//Tracking/IR Camera ==

== system top_level_arch/Manufacturing /Available Components/Avionics Package/Target Identification//Tracking/Radar Seeker ==

== system top_level_arch/Manufacturing /Available Components/Avionics Package/Viewport/ALON ==

== system top_level_arch/Manufacturing /Available Components/Avionics Package/Viewport/Sapphire ==

== system top_level_arch/Manufacturing /Available Components/Materials/Structural Material/ALON ==

== system top_level_arch/Manufacturing /Available Components/Materials/Structural Material/Inconel ==

== system top_level_arch/Manufacturing /Available Components/Materials/Structural Material/Stainless Steel ==

== system top_level_arch/Manufacturing /Available Components/Materials/Structural Material/Titantium ==

== system top_level_arch/Manufacturing /Available Components/Materials/Thermal Material/AeroTape ==

== system top_level_arch/Manufacturing /Available Components/Materials/Thermal Material/Carbon Ablators ==

== system top_level_arch/Manufacturing /Available Components/Avionics Package/Guidance Package/Dive Package/DISMAC ==

== system top_level_arch/Manufacturing /Available Components/Avionics Package/Guidance Package/Dive Package/GPS ==

== system top_level_arch/Manufacturing /Available Components/Avionics Package/Guidance Package/Dive Package/IMU ==

== system top_level_arch/Manufacturing /Available Components/Avionics Package/Guidance Package/Dive Package/STAR Tracker ==

== system top_level_arch/Manufacturing /Available Components/Avionics Package/Guidance Package/LLI Package/DISMAC ==

== system top_level_arch/Manufacturing /Available Components/Avionics Package/Guidance Package/LLI Package/GPS ==

== system top_level_arch/Manufacturing /Available Components/Avionics Package/Guidance Package/LLI Package/IMU ==

== system top_level_arch/Manufacturing /Available Components/Avionics Package/Guidance Package/LLI Package/STAR Tracker ==

== system top_level_arch/Manufacturing /Available Components/Avionics Package/Guidance Package/LLI Package/TARCOM ==
